simulink model "double_integrator_formation_control"  (R2024a)
settings: Solver=VariableStepAuto  StartTime=0.0  StopTime=5  RelTol=1e-3
settings Model: Creator=LOQ  LastModifiedBy=LOQ

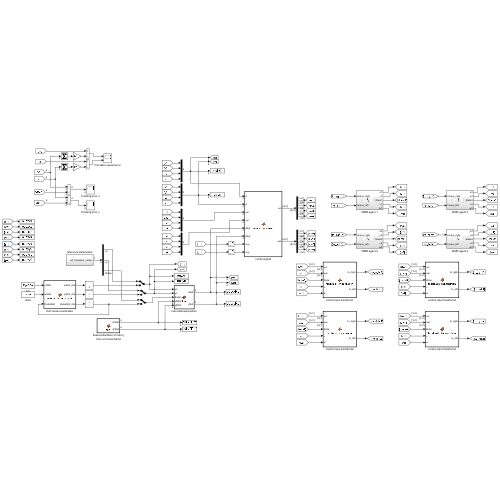
[thumbnail: Simulink's stored preview of the top-level diagram]
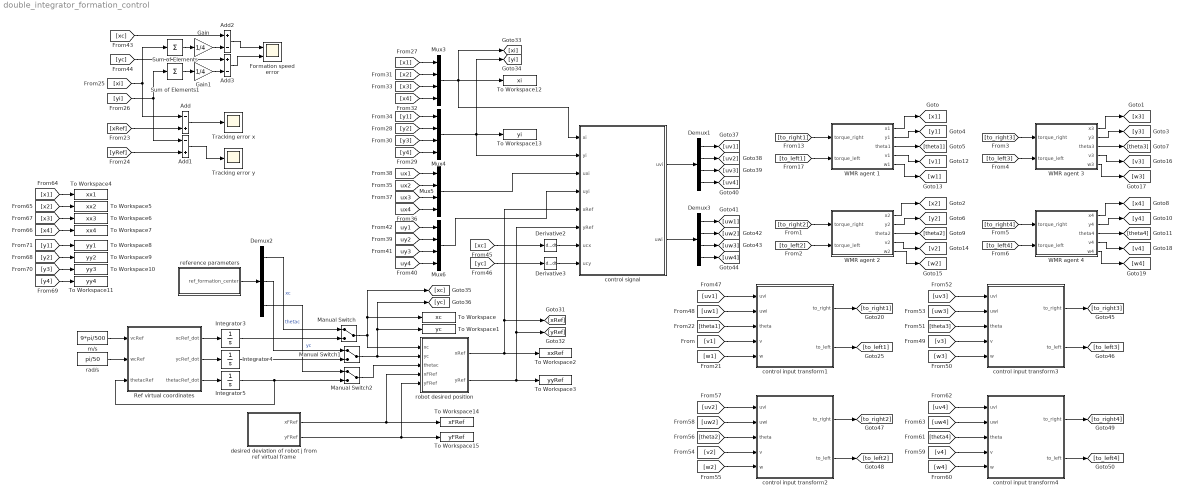
== system double_integrator_formation_control ==
  Add : Sum  Inputs=-+
  Add1 : Sum  Inputs=-+
  Add2 : Sum  Inputs=+-
  Add3 : Sum  Inputs=+-
  Demux1 : Demux
  Demux2 : Demux  Outputs=3
  Demux3 : Demux
  Derivative2 : Derivative
  Derivative3 : Derivative
  Formation speed error : Scope  NumInputPorts=2
  Gain : Gain  Gain=1/4
  Gain1 : Gain  Gain=1/4
  Integrator3 : Integrator
  Integrator4 : Integrator
  Integrator5 : Integrator
  Manual Switch : ManualSwitch
  Manual Switch1 : ManualSwitch
  Manual Switch2 : ManualSwitch
  Mux{3..6} (4 alike) : Mux
  Ref virtual coordinates : MATLAB Function  TreatAsAtomicUnit=on
  Sum of Elements : Sum  Inputs=+
  Sum of Elements1 : Sum  Inputs=+
  To Workspace : ToWorkspace  VariableName=xc  SampleTime=-1
  To Workspace1 : ToWorkspace  VariableName=yc  SampleTime=-1
  To Workspace10 : ToWorkspace  VariableName=yy3  SampleTime=-1
  To Workspace11 : ToWorkspace  VariableName=yy4  SampleTime=-1
  To Workspace12 : ToWorkspace  VariableName=xi  SampleTime=-1
  To Workspace13 : ToWorkspace  VariableName=yi  SampleTime=-1
  To Workspace14 : ToWorkspace  VariableName=xFRef  SampleTime=-1
  To Workspace15 : ToWorkspace  VariableName=yFRef  SampleTime=-1
  To Workspace2 : ToWorkspace  VariableName=xxRef  SampleTime=-1
  To Workspace3 : ToWorkspace  VariableName=yyRef  SampleTime=-1
  To Workspace4 : ToWorkspace  VariableName=xx1  SampleTime=-1
  To Workspace5 : ToWorkspace  VariableName=xx2  SampleTime=-1
  To Workspace6 : ToWorkspace  VariableName=xx3  SampleTime=-1
  To Workspace7 : ToWorkspace  VariableName=xx4  SampleTime=-1
  To Workspace8 : ToWorkspace  VariableName=yy1  SampleTime=-1
  To Workspace9 : ToWorkspace  VariableName=yy2  SampleTime=-1
  Tracking error x : Scope
  Tracking error y : Scope
  WMR agent 1 : Subsystem
  WMR agent 2 : Subsystem
  WMR agent 3 : Subsystem
  WMR agent 4 : Subsystem
  control input transform1 : MATLAB Function  TreatAsAtomicUnit=on
  control input transform2 : MATLAB Function  TreatAsAtomicUnit=on
  control input transform3 : MATLAB Function  TreatAsAtomicUnit=on
  control input transform4 : MATLAB Function  TreatAsAtomicUnit=on
  control signal : MATLAB Function  TreatAsAtomicUnit=on
  desired deviation of robot j from ref virtual frame : MATLAB Function  TreatAsAtomicUnit=on
  m/s : Constant  Value=9*pi/500
  rad/s : Constant  Value=pi/50
  reference parameters : Subsystem
  robot desired position : MATLAB Function  TreatAsAtomicUnit=on
  wires:
  Demux2/3 -> Manual Switch2/1  "thetac"
  [yc] -> Derivative3/1
  robot desired position/2(yRef) -> To Workspace3/1, control signal/6(yRef), [yRef]
  Gain/1 -> Add2/2
  [xc] -> Derivative2/1
  Manual Switch/1 -> To Workspace/1, [xc], robot desired position/1(xc)
  Mux4/1 -> [yi], To Workspace13/1, control signal/2(yi)
  [yRef] -> Add1/2
  [xi] -> Sum of Elements/1, Add/1
  [x4] -> Mux3/4
  [yc] -> Add3/1
  Sum of Elements/1 -> Gain/1
  Demux2/2 -> Manual Switch1/1  "yc"
  [to_left4] -> WMR agent 4/2(torque_left)
  m/s/1 -> Ref virtual coordinates/1(vcRef)
  [xc] -> Add2/1
  Mux6/1 -> control signal/4(uyi)
  Gain1/1 -> Add3/2
  WMR agent 4/3(theta4) -> [theta4]
  [uy2] -> Mux6/2
  [to_right4] -> WMR agent 4/1(torque_right)
  Derivative3/1 -> control signal/8(ucy)
  [yi] -> Add1/1, Sum of Elements1/1
  WMR agent 2/4(v2) -> [v2]
  Sum of Elements1/1 -> Gain1/1
  Add3/1 -> Formation speed error/2
  Add1/1 -> Tracking error y/1
  WMR agent 1/1(x1) -> [x1]
  WMR agent 4/2(y4) -> [y4]
  WMR agent 2/1(x2) -> [x2]
  [xRef] -> Add/2
  Add2/1 -> Formation speed error/1
  [theta1] -> control input transform1/3(theta)
  [x1] -> Mux3/1
  Integrator3/1 -> Manual Switch/2
  Demux2/1 -> Manual Switch/1  "xc"
  [ux3] -> Mux5/3
  reference parameters/1(ref_formation_center) -> Demux2/1
  [y4] -> Mux4/4
  WMR agent 3/5(w3) -> [w3]
  [uy1] -> Mux6/1
  [ux4] -> Mux5/4
  Mux5/1 -> control signal/3(uxi)
  [to_right2] -> WMR agent 2/1(torque_right)
  [ux1] -> Mux5/1
  [uy3] -> Mux6/3
  Ref virtual coordinates/1(xcRef_dot) -> Integrator3/1
  [uy4] -> Mux6/4
  WMR agent 1/2(y1) -> [y1]
  [x2] -> Mux3/2
  [y3] -> Mux4/3
  Integrator5/1 -> Manual Switch2/2, Ref virtual coordinates/3(thetacRef)
  [x3] -> Mux3/3
  Ref virtual coordinates/2(ycRef_dot) -> Integrator4/1
  rad/s/1 -> Ref virtual coordinates/2(wcRef)
  [y2] -> Mux4/2
  WMR agent 3/2(y3) -> [y3]
  Add/1 -> Tracking error x/1
  desired deviation of robot j from ref virtual frame/1(xFRef) -> To Workspace14/1, robot desired position/4(xFRef)
  [v1] -> control input transform1/4(v)
  Manual Switch1/1 -> [yc], To Workspace1/1, robot desired position/2(yc)
  [to_left1] -> WMR agent 1/2(torque_left)
  Integrator4/1 -> Manual Switch1/2
  WMR agent 4/1(x4) -> [x4]
  desired deviation of robot j from ref virtual frame/2(yFRef) -> To Workspace15/1, robot desired position/5(yFRef)
  [ux2] -> Mux5/2
  WMR agent 2/5(w2) -> [w2]
  WMR agent 1/3(theta1) -> [theta1]
  Mux3/1 -> [xi], To Workspace12/1, control signal/1(xi)
  WMR agent 1/5(w1) -> [w1]
  WMR agent 1/4(v1) -> [v1]
  WMR agent 4/5(w4) -> [w4]
  control signal/1(uvi) -> Demux1/1
  WMR agent 3/4(v3) -> [v3]
  [to_left3] -> WMR agent 3/2(torque_left)
  WMR agent 3/3(theta3) -> [theta3]
  [w1] -> control input transform1/5(w)
  Ref virtual coordinates/3(thetacRef_dot) -> Integrator5/1
  [y1] -> Mux4/1
  WMR agent 2/2(y2) -> [y2]
  WMR agent 4/4(v4) -> [v4]
  [to_left2] -> WMR agent 2/2(torque_left)
  robot desired position/1(xRef) -> To Workspace2/1, control signal/5(xRef), [xRef]
  WMR agent 3/1(x3) -> [x3]
  Derivative2/1 -> control signal/7(ucx)
  WMR agent 2/3(theta2) -> [theta2]
  [to_right3] -> WMR agent 3/1(torque_right)
  [to_right1] -> WMR agent 1/1(torque_right)
  control signal/2(uwi) -> Demux3/1
  Demux1/1 -> [uv1]
  Demux1/2 -> [uv2]
  Demux1/3 -> [uv3]
  Demux1/4 -> [uv4]
  Demux3/1 -> [uw1]
  Demux3/2 -> [uw2]
  Demux3/3 -> [uw3]
  Demux3/4 -> [uw4]
  [uv1] -> control input transform1/1(uvi)
  [uw1] -> control input transform1/2(uwi)
  control input transform1/1(to_right) -> [to_right1]
  control input transform1/2(to_left) -> [to_left1]
  control input transform3/2(to_left) -> [to_left3]
  control input transform3/1(to_right) -> [to_right3]
  [uw3] -> control input transform3/2(uwi)
  [uv3] -> control input transform3/1(uvi)
  [w3] -> control input transform3/5(w)
  [v3] -> control input transform3/4(v)
  [theta3] -> control input transform3/3(theta)
  [theta2] -> control input transform2/3(theta)
  [v2] -> control input transform2/4(v)
  [w2] -> control input transform2/5(w)
  [uv2] -> control input transform2/1(uvi)
  [uw2] -> control input transform2/2(uwi)
  control input transform2/1(to_right) -> [to_right2]
  control input transform2/2(to_left) -> [to_left2]
  control input transform4/2(to_left) -> [to_left4]
  control input transform4/1(to_right) -> [to_right4]
  [uw4] -> control input transform4/2(uwi)
  [uv4] -> control input transform4/1(uvi)
  [w4] -> control input transform4/5(w)
  [v4] -> control input transform4/4(v)
  [theta4] -> control input transform4/3(theta)
  Manual Switch2/1 -> robot desired position/3(thetac)
  [x3] -> To Workspace6/1
  [x2] -> To Workspace5/1
  [x1] -> To Workspace4/1
  [x4] -> To Workspace7/1
  [y3] -> To Workspace10/1
  [y1] -> To Workspace8/1
  [y2] -> To Workspace9/1
  [y4] -> To Workspace11/1

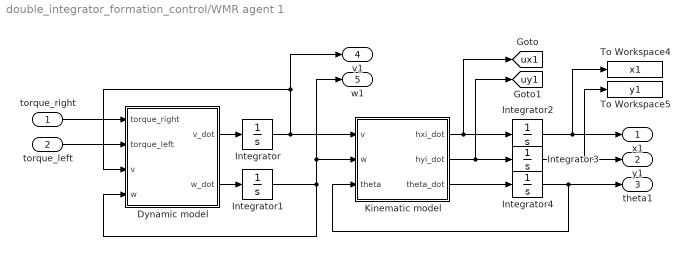
== system double_integrator_formation_control/WMR agent 1 ==
  torque_right : Inport
  torque_left : Inport  Port=2
  Dynamic model : MATLAB Function  TreatAsAtomicUnit=on
  Integrator : Integrator
  Integrator1 : Integrator
  Integrator2 : Integrator  InitialCondition=0.7
  Integrator3 : Integrator  InitialCondition=0.5
  Integrator4 : Integrator
  Kinematic model : MATLAB Function  TreatAsAtomicUnit=on
  To Workspace4 : ToWorkspace  VariableName=x1  SampleTime=-1
  To Workspace5 : ToWorkspace  VariableName=y1  SampleTime=-1
  x1 : Outport
  y1 : Outport  Port=2
  theta1 : Outport  Port=3
  v1 : Outport  Port=4
  w1 : Outport  Port=5
  tag scope: ux1=global, uy1=global
  wires:
  Dynamic model/1(v_dot) -> Integrator/1
  Integrator4/1 -> Kinematic model/3(theta), theta1/1
  Integrator1/1 -> w1/1, Kinematic model/2(w), Dynamic model/4(w)
  Integrator3/1 -> y1/1, To Workspace5/1
  torque_right/1 -> Dynamic model/1(torque_right)
  Integrator2/1 -> x1/1, To Workspace4/1
  Kinematic model/2(hyi_dot) -> [uy1], Integrator3/1
  Dynamic model/2(w_dot) -> Integrator1/1
  Integrator/1 -> Kinematic model/1(v), v1/1, Dynamic model/3(v)
  Kinematic model/3(theta_dot) -> Integrator4/1
  Kinematic model/1(hxi_dot) -> [ux1], Integrator2/1
  torque_left/1 -> Dynamic model/2(torque_left)

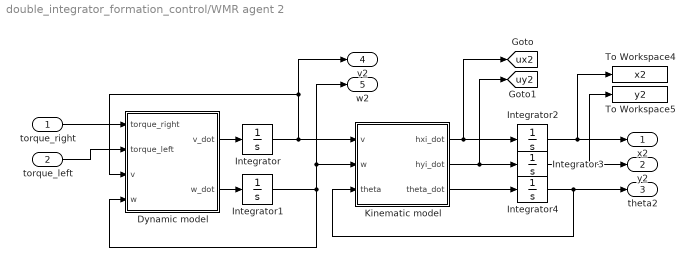
== system double_integrator_formation_control/WMR agent 2 ==
  torque_right : Inport
  torque_left : Inport  Port=2
  Dynamic model : MATLAB Function  TreatAsAtomicUnit=on
  Integrator : Integrator
  Integrator1 : Integrator
  Integrator2 : Integrator  InitialCondition=-0.6
  Integrator3 : Integrator  InitialCondition=0.4
  Integrator4 : Integrator  InitialCondition=pi/2
  Kinematic model : MATLAB Function  TreatAsAtomicUnit=on
  To Workspace4 : ToWorkspace  VariableName=x2  SampleTime=-1
  To Workspace5 : ToWorkspace  VariableName=y2  SampleTime=-1
  x2 : Outport
  y2 : Outport  Port=2
  theta2 : Outport  Port=3
  v2 : Outport  Port=4
  w2 : Outport  Port=5
  tag scope: ux2=global, uy2=global
  wires:
  Dynamic model/1(v_dot) -> Integrator/1
  Integrator4/1 -> theta2/1, Kinematic model/3(theta)
  Integrator1/1 -> Kinematic model/2(w), w2/1, Dynamic model/4(w)
  Integrator3/1 -> y2/1, To Workspace5/1
  torque_right/1 -> Dynamic model/1(torque_right)
  Integrator2/1 -> x2/1, To Workspace4/1
  Kinematic model/2(hyi_dot) -> [uy2], Integrator3/1
  Dynamic model/2(w_dot) -> Integrator1/1
  Integrator/1 -> v2/1, Dynamic model/3(v), Kinematic model/1(v)
  Kinematic model/3(theta_dot) -> Integrator4/1
  Kinematic model/1(hxi_dot) -> [ux2], Integrator2/1
  torque_left/1 -> Dynamic model/2(torque_left)

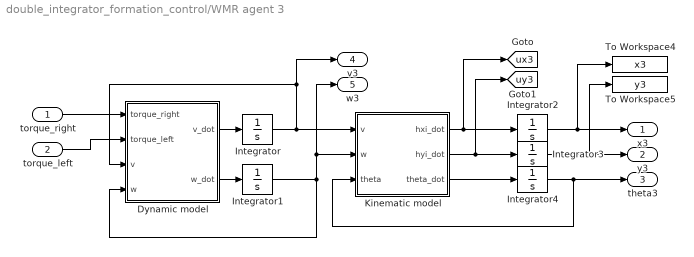
== system double_integrator_formation_control/WMR agent 3 ==
  torque_right : Inport
  torque_left : Inport  Port=2
  Dynamic model : MATLAB Function  TreatAsAtomicUnit=on
  Integrator : Integrator
  Integrator1 : Integrator
  Integrator2 : Integrator  InitialCondition=-0.8
  Integrator3 : Integrator  InitialCondition=0.3
  Integrator4 : Integrator  InitialCondition=-pi/3
  Kinematic model : MATLAB Function  TreatAsAtomicUnit=on
  To Workspace4 : ToWorkspace  VariableName=x3  SampleTime=-1
  To Workspace5 : ToWorkspace  VariableName=y3  SampleTime=-1
  x3 : Outport
  y3 : Outport  Port=2
  theta3 : Outport  Port=3
  v3 : Outport  Port=4
  w3 : Outport  Port=5
  tag scope: ux3=global, uy3=global
  wires:
  Dynamic model/1(v_dot) -> Integrator/1
  Integrator4/1 -> theta3/1, Kinematic model/3(theta)
  Integrator1/1 -> w3/1, Kinematic model/2(w), Dynamic model/4(w)
  Integrator3/1 -> y3/1, To Workspace5/1
  torque_right/1 -> Dynamic model/1(torque_right)
  Integrator2/1 -> x3/1, To Workspace4/1
  Dynamic model/2(w_dot) -> Integrator1/1
  Integrator/1 -> Kinematic model/1(v), v3/1, Dynamic model/3(v)
  Kinematic model/3(theta_dot) -> Integrator4/1
  Kinematic model/1(hxi_dot) -> [ux3], Integrator2/1
  torque_left/1 -> Dynamic model/2(torque_left)
  Kinematic model/2(hyi_dot) -> [uy3], Integrator3/1

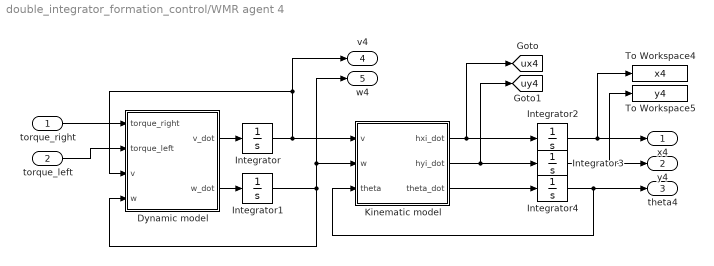
== system double_integrator_formation_control/WMR agent 4 ==
  torque_right : Inport
  torque_left : Inport  Port=2
  Dynamic model : MATLAB Function  TreatAsAtomicUnit=on
  Integrator : Integrator
  Integrator1 : Integrator
  Integrator2 : Integrator  InitialCondition=-0.5
  Integrator3 : Integrator  InitialCondition=0.9
  Integrator4 : Integrator  InitialCondition=pi/4
  Kinematic model : MATLAB Function  TreatAsAtomicUnit=on
  To Workspace4 : ToWorkspace  VariableName=x4  SampleTime=-1
  To Workspace5 : ToWorkspace  VariableName=y4  SampleTime=-1
  x4 : Outport
  y4 : Outport  Port=2
  theta4 : Outport  Port=3
  v4 : Outport  Port=4
  w4 : Outport  Port=5
  tag scope: ux4=global, uy4=global
  wires:
  Dynamic model/1(v_dot) -> Integrator/1
  Integrator4/1 -> theta4/1, Kinematic model/3(theta)
  Integrator1/1 -> w4/1, Kinematic model/2(w), Dynamic model/4(w)
  Integrator3/1 -> y4/1, To Workspace5/1
  torque_right/1 -> Dynamic model/1(torque_right)
  Integrator2/1 -> x4/1, To Workspace4/1
  Kinematic model/2(hyi_dot) -> [uy4], Integrator3/1
  Dynamic model/2(w_dot) -> Integrator1/1
  Integrator/1 -> Kinematic model/1(v), v4/1, Dynamic model/3(v)
  Kinematic model/3(theta_dot) -> Integrator4/1
  Kinematic model/1(hxi_dot) -> [ux4], Integrator2/1
  torque_left/1 -> Dynamic model/2(torque_left)

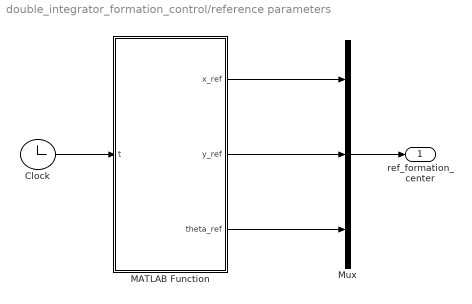
== system double_integrator_formation_control/reference parameters ==
  Clock : Clock
  MATLAB Function : MATLAB Function  TreatAsAtomicUnit=on
  Mux : Mux  Inputs=3
  ref_formation_center : Outport
  wires:
  Mux/1 -> ref_formation_center/1
  Clock/1 -> MATLAB Function/1(t)
  MATLAB Function/1(x_ref) -> Mux/1
  MATLAB Function/2(y_ref) -> Mux/2
  MATLAB Function/3(theta_ref) -> Mux/3

== matlab function double_integrator_formation_control/control signal ==
  data: uvi output; uwi output; xi input; yi input; uxi input; uyi input; xRef input; yRef input; ucx input; ucy input
function [uvi, uwi] = consensus_algo(xi, yi, uxi, uyi, xRef, yRef, ucx, ucy)

A = [0 1 1 0;
     1 0 0 1;
     0 1 0 0;
     1 0 1 0];
D = diag([2, 2, 1, 2]);
alpha1 = 60;
alpha2 = 60;
alpha3 = 60;
alpha4 = 60;
Q = diag([alpha1, alpha2, alpha3, alpha4]);
L = D - A;

% k1 = 4;    
% k2 = 30;
% 
% uvi = - k1*(L+Q)*(xi-xRef) - k2*(uxi-ucx);
% uwi = - k1*(L+Q)*(yi-yRef) - k2*(uyi-ucy);


k2 = 120;
k1 = 600;
uvi = -(k1*eye(4)+L)*(xi-xRef) -k2*(uxi-ucx);
uwi = -(k1*eye(4)+L)*(yi-yRef) -k2*(uyi-ucy);

end

== matlab function double_integrator_formation_control/control input transform1 ==
  data: uvi input; uwi input; to_right output; to_left output; theta input; v input; w input
function [to_right, to_left] = feedback_linearization(uvi,uwi,theta,v,w)

a = 0.2;
mG = 10;
r = 0.15;
L = 0.6;
I_G = 4;


% V_dot = B*V + N*To
% The goal is to make p_dot_dot = u
% u = p_dot_dot = S_dot*V+S*V_dot = (S_dot+S*B)*V + S*N*To

S = [cos(theta) -a*sin(theta);
     sin(theta) a*cos(theta)];
S_dot = [-w*sin(theta) -a*w*cos(theta);
     w*cos(theta) -a*w*sin(theta)];
B = [0 a*w;
     -mG*a*w/(I_G+mG*a^2) 0];
N = [1/(mG*r) 1/(mG*r);
     L/(2*r*(I_G+mG*a^2)) -L/(2*r*(I_G+mG*a^2))];

V = [v;w];
u = [uvi;uwi];

To = N\(S\( u - (S_dot+S*B)*V));
to_right = To(1);
to_left = To(2);

end

== matlab function double_integrator_formation_control/WMR agent 4/Dynamic model ==
  data: torque_right input; v_dot output; torque_left input; v input; w input; w_dot output
function [v_dot , w_dot] = Dynamic(torque_right , torque_left, v, w)

a = 0.2;
mG = 10;
r = 0.15;
L = 0.6;
I_G = 4;

% V matrix 
V = [v ; w];

% Torque matrix
To = [torque_right ; torque_left];

B = [0 a*w;
     -mG*a*w/(I_G+mG*a^2) 0];
N = [1/(mG*r) 1/(mG*r);
     L/(2*r*(I_G+mG*a^2)) -L/(2*r*(I_G+mG*a^2))];

V_dot = B*V + N*To;
v_dot = V_dot(1);
w_dot = V_dot(2);

end

== matlab function double_integrator_formation_control/WMR agent 4/Kinematic model ==
  data: v input; hxi_dot output; w input; theta input; hyi_dot output; theta_dot output
function [hxi_dot, hyi_dot, theta_dot] = Kinematic (v,w,theta)

a = 0.2;
R = [cos(theta) -a*sin(theta);
     sin(theta) a*cos(theta);
     0 1];

V = [v; w];

% Output
H = R*V;

hxi_dot = H(1);
hyi_dot = H(2);
theta_dot = H(3);

end

== matlab function double_integrator_formation_control/desired deviation of robot j from ref virtual frame ==
  data: xFRef output; yFRef output
function [xFRef, yFRef] = fcn ()
% Squared formation

l = 0.6;
j = [1;2;3;4];
% phiRef = pi*[1;1;1;1] - pi/4 * j;
phiRef = pi/2 * (j-1);
xFRef = l*cos(phiRef); 
yFRef = l*sin(phiRef);
          
end

== matlab function double_integrator_formation_control/robot desired position ==
  data: xRef output; yRef output; xc input; yc input; thetac input; xFRef input; yFRef input
function [xRef, yRef] = fcn (xc, yc, thetac, xFRef, yFRef)

% R = [cos(thetac) -sin(thetac);
%      sin(thetac) cos(thetac)];
% rF = [xFRef; yFRef];
% rc = [xc; yc];
% Q = rc + R*rF;
% 
% xRef = Q(1); 
% yRef = Q(2);
          
xRef = xc*[1;1;1;1] + cos(thetac)*xFRef - sin(thetac)*yFRef;
yRef = yc*[1;1;1;1] + sin(thetac)*xFRef + cos(thetac)*yFRef;

% xRef = xc+xFRef;
% yRef = yc+yFRef;
end

== matlab function double_integrator_formation_control/reference parameters/MATLAB Function ==
  data: x_ref output; y_ref output; theta_ref output; t input
function [x_ref,y_ref,theta_ref] = reference(t)

% Curved trajectory
% w = pi/6;
% x_ref = 3*sin(w*t);
% y_ref = 3*cos(w*t);
% dxRef = 3*w*cos(w*t);
% dyRef =  -3*w*sin(w*t);
% theta_ref =  atan2(dyRef, dxRef);

% curved trajectory
x_ref = -t;
y_ref = sin(0.5*t)+0.5*t+1;
dxRef = -1;
dyRef =  0.5*cos(0.5*t)+0.5;
theta_ref =  atan2(dyRef, dxRef);


end

== matlab function double_integrator_formation_control/control input transform3 ==
  data: uvi input; uwi input; to_right output; to_left output; theta input; v input; w input
function [to_right, to_left] = feedback_linearization(uvi,uwi,theta,v,w)

a = 0.2;
mG = 10;
r = 0.15;
L = 0.6;
I_G = 4;


% V_dot = B*V + N*To
% The goal is to make p_dot_dot = u
% u = p_dot_dot = S_dot*V+S*V_dot = (S_dot+S*B)*V + S*N*To

S = [cos(theta) -a*sin(theta);
     sin(theta) a*cos(theta)];
S_dot = [-w*sin(theta) -a*w*cos(theta);
     w*cos(theta) -a*w*sin(theta)];
B = [0 a*w;
     -mG*a*w/(I_G+mG*a^2) 0];
N = [1/(mG*r) 1/(mG*r);
     L/(2*r*(I_G+mG*a^2)) -L/(2*r*(I_G+mG*a^2))];

V = [v;w];
u = [uvi;uwi];

To = N\(S\( u - (S_dot+S*B)*V));
to_right = To(1);
to_left = To(2);

end

== matlab function double_integrator_formation_control/control input transform2 ==
  data: uvi input; uwi input; to_right output; to_left output; theta input; v input; w input
function [to_right, to_left] = feedback_linearization(uvi,uwi,theta,v,w)

a = 0.2;
mG = 10;
r = 0.15;
L = 0.6;
I_G = 4;


% V_dot = B*V + N*To
% The goal is to make p_dot_dot = u
% u = p_dot_dot = S_dot*V+S*V_dot = (S_dot+S*B)*V + S*N*To

S = [cos(theta) -a*sin(theta);
     sin(theta) a*cos(theta)];
S_dot = [-w*sin(theta) -a*w*cos(theta);
     w*cos(theta) -a*w*sin(theta)];
B = [0 a*w;
     -mG*a*w/(I_G+mG*a^2) 0];
N = [1/(mG*r) 1/(mG*r);
     L/(2*r*(I_G+mG*a^2)) -L/(2*r*(I_G+mG*a^2))];

V = [v;w];
u = [uvi;uwi];

To = N\(S\( u - (S_dot+S*B)*V));
to_right = To(1);
to_left = To(2);

end

== matlab function double_integrator_formation_control/control input transform4 ==
  data: uvi input; uwi input; to_right output; to_left output; theta input; v input; w input
function [to_right, to_left] = feedback_linearization(uvi,uwi,theta,v,w)

a = 0.2;
mG = 10;
r = 0.15;
L = 0.6;
I_G = 4;


% V_dot = B*V + N*To
% The goal is to make p_dot_dot = u
% u = p_dot_dot = S_dot*V+S*V_dot = (S_dot+S*B)*V + S*N*To

S = [cos(theta) -a*sin(theta);
     sin(theta) a*cos(theta)];
S_dot = [-w*sin(theta) -a*w*cos(theta);
     w*cos(theta) -a*w*sin(theta)];
B = [0 a*w;
     -mG*a*w/(I_G+mG*a^2) 0];
N = [1/(mG*r) 1/(mG*r);
     L/(2*r*(I_G+mG*a^2)) -L/(2*r*(I_G+mG*a^2))];

V = [v;w];
u = [uvi;uwi];

To = N\(S\( u - (S_dot+S*B)*V));
to_right = To(1);
to_left = To(2);

end

== matlab function double_integrator_formation_control/WMR agent 1/Dynamic model ==
  data: torque_right input; v_dot output; torque_left input; v input; w input; w_dot output
function [v_dot , w_dot] = Dynamic(torque_right , torque_left, v, w)

a = 0.2;
mG = 10;
r = 0.15;
L = 0.6;
I_G = 4;

% V matrix 
V = [v ; w];

% Torque matrix
To = [torque_right ; torque_left];

B = [0 a*w;
     -mG*a*w/(I_G+mG*a^2) 0];
N = [1/(mG*r) 1/(mG*r);
     L/(2*r*(I_G+mG*a^2)) -L/(2*r*(I_G+mG*a^2))];

V_dot = B*V + N*To;
v_dot = V_dot(1);
w_dot = V_dot(2);

end

== matlab function double_integrator_formation_control/WMR agent 1/Kinematic model ==
  data: v input; hxi_dot output; w input; theta input; hyi_dot output; theta_dot output
function [hxi_dot, hyi_dot, theta_dot] = Kinematic (v,w,theta)

a = 0.2;
R = [cos(theta) -a*sin(theta);
     sin(theta) a*cos(theta);
     0 1];

V = [v; w];

% Output
H = R*V;

hxi_dot = H(1);
hyi_dot = H(2);
theta_dot = H(3);

end

== matlab function double_integrator_formation_control/WMR agent 2/Dynamic model ==
  data: torque_right input; v_dot output; torque_left input; v input; w input; w_dot output
function [v_dot , w_dot] = Dynamic(torque_right , torque_left, v, w)

a = 0.2;
mG = 10;
r = 0.15;
L = 0.6;
I_G = 4;

% V matrix 
V = [v ; w];

% Torque matrix
To = [torque_right ; torque_left];

B = [0 a*w;
     -mG*a*w/(I_G+mG*a^2) 0];
N = [1/(mG*r) 1/(mG*r);
     L/(2*r*(I_G+mG*a^2)) -L/(2*r*(I_G+mG*a^2))];

V_dot = B*V + N*To;
v_dot = V_dot(1);
w_dot = V_dot(2);

end

== matlab function double_integrator_formation_control/WMR agent 2/Kinematic model ==
  data: v input; hxi_dot output; w input; theta input; hyi_dot output; theta_dot output
function [hxi_dot, hyi_dot, theta_dot] = Kinematic (v,w,theta)

a = 0.2;
R = [cos(theta) -a*sin(theta);
     sin(theta) a*cos(theta);
     0 1];

V = [v; w];

% Output
H = R*V;

hxi_dot = H(1);
hyi_dot = H(2);
theta_dot = H(3);

end

== matlab function double_integrator_formation_control/WMR agent 3/Dynamic model ==
  data: torque_right input; v_dot output; torque_left input; v input; w input; w_dot output
function [v_dot , w_dot] = Dynamic(torque_right , torque_left, v, w)

a = 0.2;
mG = 10;
r = 0.15;
L = 0.6;
I_G = 4;

% V matrix 
V = [v ; w];

% Torque matrix
To = [torque_right ; torque_left];

B = [0 a*w;
     -mG*a*w/(I_G+mG*a^2) 0];
N = [1/(mG*r) 1/(mG*r);
     L/(2*r*(I_G+mG*a^2)) -L/(2*r*(I_G+mG*a^2))];

V_dot = B*V + N*To;
v_dot = V_dot(1);
w_dot = V_dot(2);

end

== matlab function double_integrator_formation_control/WMR agent 3/Kinematic model ==
  data: v input; hxi_dot output; w input; theta input; hyi_dot output; theta_dot output
function [hxi_dot, hyi_dot, theta_dot] = Kinematic (v,w,theta)

a = 0.2;
R = [cos(theta) -a*sin(theta);
     sin(theta) a*cos(theta);
     0 1];

V = [v; w];

% Output
H = R*V;

hxi_dot = H(1);
hyi_dot = H(2);
theta_dot = H(3);

end

== matlab function double_integrator_formation_control/Ref virtual coordinates ==
  data: vcRef input; xcRef_dot output; wcRef input; thetacRef input; ycRef_dot output; thetacRef_dot output
function [xcRef_dot, ycRef_dot, thetacRef_dot] = center_of_formation (vcRef,wcRef,thetacRef)

R = [cos(thetacRef) 0;
     sin(thetacRef) 0;
      0 1];
V = [vcRef; wcRef];

Q = R*V;

xcRef_dot = Q(1); 
ycRef_dot = Q(2);
thetacRef_dot = Q(3);           

end
